simulink model "model"  (R2020b)
settings: Solver=ode15s  StartTime=0.0  StopTime=1e5  RelTol=1e-8  AbsTol=1e-8
libraries: libraryMatlab x4
settings Model: Creator=pacif  LastModifiedBy=pacif

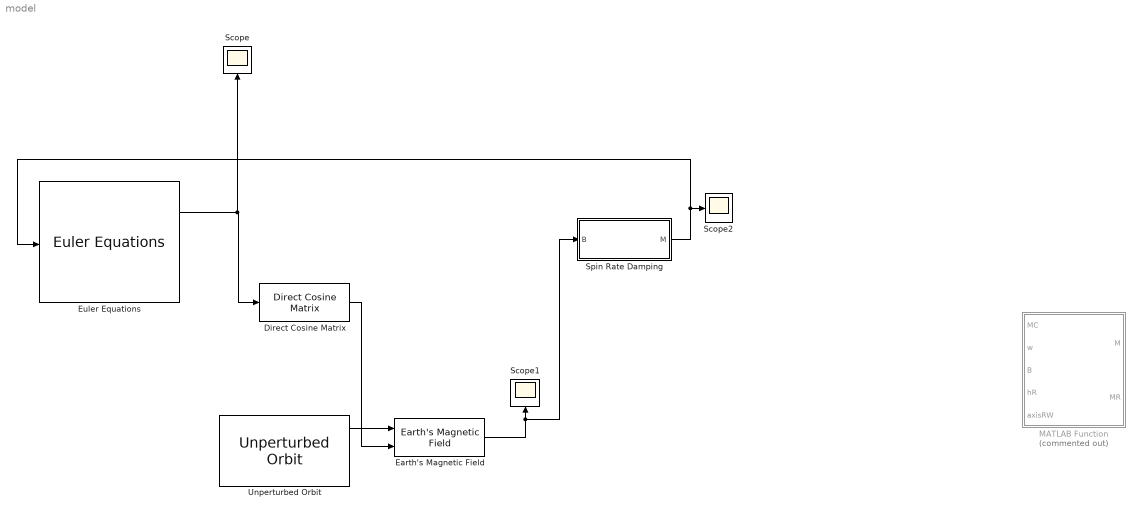
== system model ==
  Direct Cosine Matrix : libraryMatlab/Direct Cosine Matrix  SystemSampleTime=-1  VariantActivationTime=update diagram  Latency=0  AutoFrameSizeCalculation=off
  Earth's Magnetic Field : libraryMatlab/Earth's Magnetic Field  SystemSampleTime=-1  VariantActivationTime=update diagram  Latency=0  AutoFrameSizeCalculation=off
  Euler Equations : libraryMatlab/Euler Equations  SystemSampleTime=-1  VariantActivationTime=update diagram  Latency=0  AutoFrameSizeCalculation=off
  MATLAB Function : MATLAB Function  Commented=on  TreatAsAtomicUnit=on
  Scope : Scope
  Scope1 : Scope
  Scope2 : Scope
  Spin Rate Damping : Subsystem  AncestorBlock=libraryMatlab/Spin Rate Damping
  Unperturbed Orbit : libraryMatlab/Unperturbed Orbit  SystemSampleTime=-1  VariantActivationTime=update diagram  Latency=0  AutoFrameSizeCalculation=off
  wires:
  Euler Equations/1 -> Direct Cosine Matrix/1, Scope/1
  Unperturbed Orbit/1 -> Earth's Magnetic Field/1
  Direct Cosine Matrix/1 -> Earth's Magnetic Field/2
  Earth's Magnetic Field/1 -> Spin Rate Damping/1(B), Scope1/1
  Spin Rate Damping/1(M) -> Scope2/1, Euler Equations/1

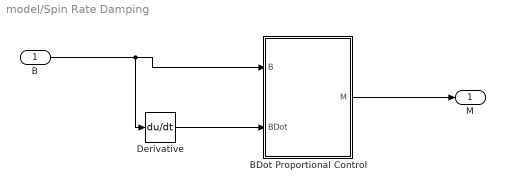
== system model/Spin Rate Damping ==
  B : Inport
  BDot Proportional Control : MATLAB Function  TreatAsAtomicUnit=on
  Derivative : Derivative  CoefficientInTFapproximation=0
  M : Outport
  wires:
  BDot Proportional Control/1(M) -> M/1
  B/1 -> Derivative/1, BDot Proportional Control/1(B)
  Derivative/1 -> BDot Proportional Control/2(BDot)

== matlab function model/MATLAB Function ==
  data: MC input; M output; w input; B input; hR input; axisRW input; MR output
function [M,MR] = fun(MC, w, B, hR, axisRW)

MC1 = MC + cross(w,hR*axisRW);

Bx = B(1); By = B(2); Bz = B(3);

% C = [0      Bz      -By     0
%     -Bz     0       Bx      0
%     By      -Bx     0       -1];
% 
% invC = pinv(C);
% 
% u = invC*MC1;
% 
% D = u(1:3)*normB; MR = u(4);
% 
% if abs(D(1)) > 140, D(1) = sign(D(1))*140; end
% if abs(D(2)) > 140, D(2) = sign(D(2))*140; end

Dx = -MC1(2)/Bz; Dy = MC1(1)/Bz;

if abs(Dx) > 140, Dx = sign(Dx)*140; end
if abs(Dy) > 140, Dy = sign(Dy)*140; end

MR = -MC1(3) + By*Dx - Bx*Dy;

if abs(MR) > 18; MR = sign(MR)*18; end
% % if hR >= 0.2 && MR > 0, MR = 0; end
% % if hR <= -0.2 && MR < 0, MR = 0; end

D = [Dx; Dy; 0]; 

M1 = cross(D,B);

M2 = -cross(w,axisRW*hR) - axisRW*MR;


M = M1 + M2;

    


end

== matlab function model/Spin Rate Damping/BDot Proportional Control ==
  data: B input; BDot input; M output
function M = fcn(B,BDot)

m0 = 140;
signBDot = sign(BDot);

m = -m0*signBDot;


M = cross(m,B);
